simulink model "ffb_Cularis_attitudeloopclosed"  (Simulink 8.6)
settings: Solver=FixedStepAuto  SolverMode=SingleTasking  StartTime=0.0  StopTime=uavsim.simConfig.tsim  FixedStep=uavsim.simConfig.tsample_model  RelTol=1
model workspace (MAT data in the model file):
  VortexSig = Simulink.Signal
  VortexSig.DataType = 'Bus: VortexStates'
  VortexSig.Units = 'auto'
  VortexSig.Dimensions = [10 1]
  VortexSig.DimensionsMode = 'Fixed'
  VortexSig.Complexity = 'real'
  VortexSig.SampleTime = -1
  VortexSig.SamplingMode = 'auto'
  VortexSig.InitialValue = 'VortexStates_MATLABStruct_array'
undefined symbols (not defined in the file or in its folder): uavsim
libraries: aerolibtransform2 x2, aerolibutil x2, aerolibanimutils x1, uavsimBlockset_Cularis_withUAV3D x1
settings Model: Creator=mstolle  LastModifiedBy=j.bolting  ExtModeTrigDuration=100
settings SolverCC: ZcThreshold=1e-5  ZeroCrossAlgorithm=Adaptive  AlgebraicLoopSolver=LineSearch  AutoInsertRateTranBlk=on
settings DataIOCC: LimitDataPoints=off  SaveFinalState=on  SaveFormat=StructureWithTime  SignalLoggingSaveFormat=Dataset  SaveOutput=off  SaveState=on  DSMLogging=off  InspectSignalLogs=on  StateSaveName=tmp_raccel_xout
settings OptimizationCC: BlockReduction=off  OptimizeBlockIOStorage=off  BufferReuse=off  GlobalBufferReuse=off  ExpressionFolding=off  LocalBlockOutputs=off  EfficientMapNaN2IntZero=off  SimCompilerOptimization=on
settings DebuggingCC: UnderspecifiedInitializationDetection=Simplified  MergeDetectMultiDrivingBlocksExec=error  IgnoredZcDiagnostic=none  FcnCallInpInsideContextMsg=EnableAllAsError  BusObjectLabelMismatch=error
settings HardwareCC: TargetBitPerPointer=64  TargetLongLongMode=on  TargetIntDivRoundTo=Zero  TargetEndianess=LittleEndian  TargetWordSize=64  TargetHWDeviceType=MATLAB Host  ProdEqTarget=off
settings ModelReferenceCC: UpdateModelReferenceTargets=IfOutOfDate  ModelReferenceNumInstancesAllowed=Single  ModelReferenceMinAlgLoopOccurrences=on
settings SFSimCC: SFSimEcho=off
settings RTWCC: SystemTargetFile=raccel.tlc  TemplateMakefile=raccel_default_tmf  RTWVerbose=off  RTWUseSimCustomCode=on
settings CodeAppCC: GenerateComments=off  MaxIdLength=128  SimulinkBlockComments=off
settings RaccelTargetCC: ERTMultiwordTypeDef=System defined  ERTMultiwordLength=256  GeneratePreprocessorConditionals=Use local settings  ERTFirstTimeCompliant=off  MultiInstanceERTCode=off  ENABLE_SLEXEC_SSBRIDGE=0  RTWCAPIParams=on
settings ConfigComp: CovSFcnEnable=off
settings ConfigurationSet: Description=SimMechanics 2G

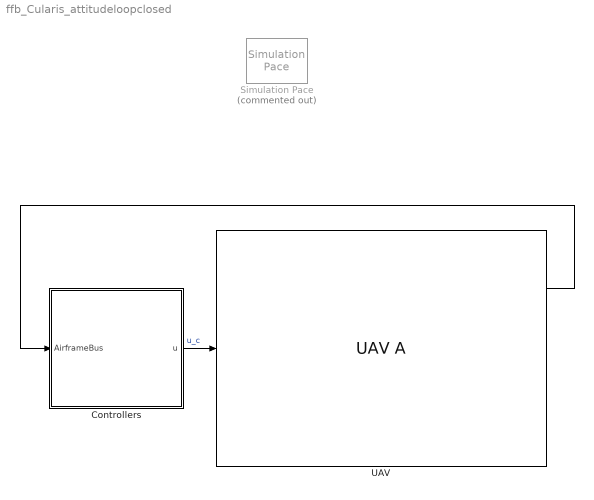
== system ffb_Cularis_attitudeloopclosed ==
  Controllers : Subsystem
  Simulation Pace : aerolibanimutils/Simulation Pace  Commented=on  SimulationPace=1  SleepMode=MATLAB Thread  OutputPaceError=off  SampleTime=-1
  UAV : uavsimBlockset_Cularis_withUAV3D/UAV A  aircraftmask_phithetapsi0=[uavsim.cularis.phithetapsi0(1:2); deg2rad(-30)]'  aircraftmask_p0_NED_m=[0 0 -50]  aircraftmask_originNED_ECEF_rrm=uavsim.originNED_ECEF_radradm  aircraftmask_pqr0=uavsim.cularis.omega0  aircraftmask_uvw0=uavsim.cularis.uvw0  aircraftmask_phithetapsi_trim=uavsim.cularis.phithetapsi0  aircraftmask_ID=1  aircraftmask_wakevortexenabled=off  aircraftmask_navigationLaw=-1  uavsim=uavsim  leaderID=0  aircraftmask_displayUAV3D=on  aircraftmask_displayVortices=off
  wires:
  UAV/1 -> Controllers/1(AirframeBus)
  Controllers/1(u) -> UAV/1  "u_c"

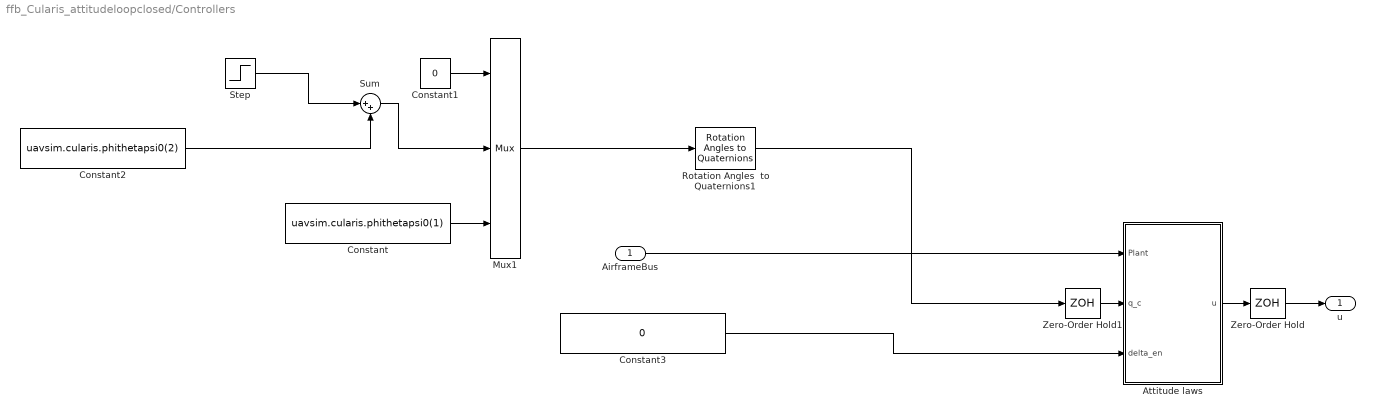
== system ffb_Cularis_attitudeloopclosed/Controllers ==
  AirframeBus : Inport
  Attitude laws : Subsystem  SystemSampleTime=uavsim.ap.hardware.dt_attitudeloops_s
  Constant : Constant  Value=uavsim.cularis.phithetapsi0(1)
  Constant1 : Constant  Value=0
  Constant2 : Constant  Value=uavsim.cularis.phithetapsi0(2)
  Constant3 : Constant  Value=0
  Mux1 : Mux  Inputs=3
  Rotation Angles  to Quaternions1 : aerolibtransform2/Rotation Angles to Quaternions  rotationOrder=ZYX
  Step : Step  Time=10  After=deg2rad(3)  SampleTime=0
  Sum : Sum  Inputs=|++
  Zero-Order Hold : ZeroOrderHold  SampleTime=uavsim.ap.tsampling_attitudelaws
  Zero-Order Hold1 : ZeroOrderHold  SampleTime=uavsim.ap.tsampling_guidancelaws
  u : Outport
  wires:
  Zero-Order Hold/1 -> u/1
  Mux1/1 -> Rotation Angles  to Quaternions1/1
  AirframeBus/1 -> Attitude laws/1(Plant)
  Attitude laws/1(u) -> Zero-Order Hold/1
  Rotation Angles  to Quaternions1/1 -> Zero-Order Hold1/1
  Zero-Order Hold1/1 -> Attitude laws/2(q_c)
  Constant1/1 -> Mux1/1
  Constant/1 -> Mux1/3
  Constant2/1 -> Sum/2
  Constant3/1 -> Attitude laws/3(delta_en)
  Step/1 -> Sum/1
  Sum/1 -> Mux1/2

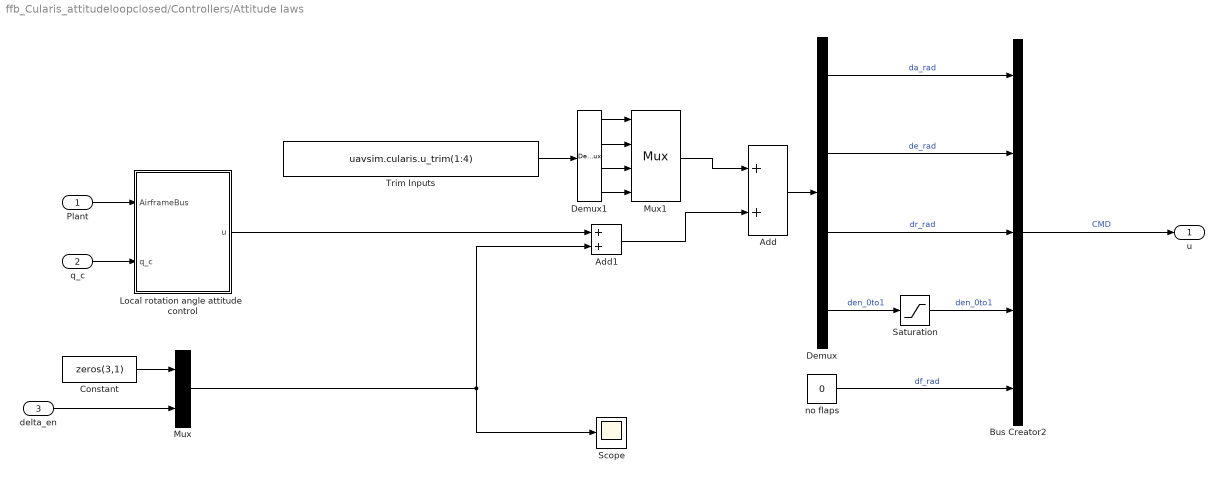
== system ffb_Cularis_attitudeloopclosed/Controllers/Attitude laws ==
  Plant : Inport  OutDataTypeStr=Bus: Airframe
  q_c : Inport  Port=2
  delta_en : Inport  Port=3
  Add : Sum
  Add1 : Sum
  Bus Creator2 : BusCreator  Inputs=5  OutDataTypeStr=Bus: CMD  NonVirtualBus=on
  Constant : Constant  Value=zeros(3,1)
  Demux : Demux
  Demux1 : Demux
  Local rotation angle attitude  control : Subsystem
  Mux : Mux  Inputs=2
  Mux1 : Mux
  Saturation : Saturate  UpperLimit=1  LowerLimit=0
  Scope : Scope
  Trim Inputs : Constant  Value=uavsim.cularis.u_trim(1:4)
  no flaps : Constant  Value=0
  u : Outport  OutDataTypeStr=Bus: CMD
  wires:
  no flaps/1 -> Bus Creator2/5  "df_rad"
  delta_en/1 -> Mux/2
  Add1/1 -> Add/2
  Mux/1 -> Scope/1, Add1/2
  Constant/1 -> Mux/1
  q_c/1 -> Local rotation angle attitude  control/2(q_c)
  Plant/1 -> Local rotation angle attitude  control/1(AirframeBus)
  Add/1 -> Demux/1
  Mux1/1 -> Add/1
  Demux/2 -> Bus Creator2/2  "de_rad"
  Demux/1 -> Bus Creator2/1  "da_rad"
  Saturation/1 -> Bus Creator2/4  "den_0to1"
  Demux/3 -> Bus Creator2/3  "dr_rad"
  Bus Creator2/1 -> u/1  "CMD"
  Local rotation angle attitude  control/1(u) -> Add1/1
  Demux/4 -> Saturation/1  "den_0to1"
  Trim Inputs/1 -> Demux1/1
  Demux1/4 -> Mux1/4
  Demux1/1 -> Mux1/1
  Demux1/3 -> Mux1/3
  Demux1/2 -> Mux1/2

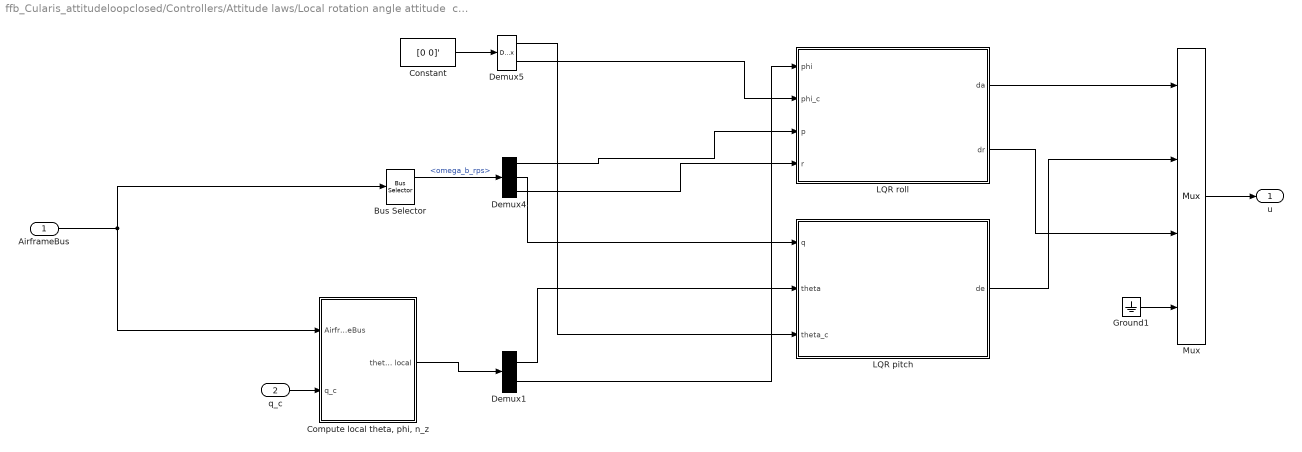
== system ffb_Cularis_attitudeloopclosed/Controllers/Attitude laws/Local rotation angle attitude  control ==
  AirframeBus : Inport  OutDataTypeStr=Bus: Airframe
  q_c : Inport  Port=2
  Bus Selector : BusSelector  OutputSignals=Kinematics.RotationalVelocity.omega_b_rps,Kinematics.Attitude.euler_rad
  "Compute local theta, phi, n_z" : Subsystem
  Constant : Constant  Value=[0 0]'
  Demux1 : Demux  Outputs=2
  Demux4 : Demux  Outputs=3
  Demux5 : Demux  Outputs=2
  Ground1 : Ground
  LQR pitch : Subsystem
  LQR roll : Subsystem
  Mux : Mux
  u : Outport
  wires:
  Ground1/1 -> Mux/4
  q_c/1 -> "Compute local theta, phi, n_z"/2(q_c)
  Mux/1 -> u/1
  Constant/1 -> Demux5/1
  Bus Selector/1 -> Demux4/1  "<omega_b_rps>"
  Demux5/2 -> LQR roll/2(phi_c)
  Demux4/1 -> LQR roll/3(p)
  Demux4/3 -> LQR roll/4(r)
  Demux5/1 -> LQR pitch/3(theta_c)
  Demux4/2 -> LQR pitch/1(q)
  LQR pitch/1(de) -> Mux/2
  LQR roll/1(da) -> Mux/1
  LQR roll/2(dr) -> Mux/3
  AirframeBus/1 -> "Compute local theta, phi, n_z"/1(AirframeBus), Bus Selector/1
  "Compute local theta, phi, n_z"/1("theta, phi local") -> Demux1/1
  Demux1/1 -> LQR pitch/2(theta)
  Demux1/2 -> LQR roll/1(phi)

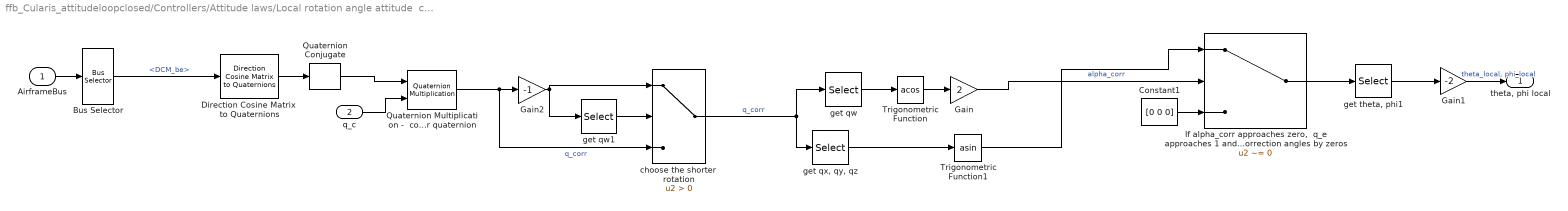
== system ffb_Cularis_attitudeloopclosed/Controllers/Attitude laws/Local rotation angle attitude  control/Compute local theta, phi, n_z ==
  AirframeBus : Inport  OutDataTypeStr=Bus: Airframe
  q_c : Inport  Port=2
  Bus Selector : BusSelector  OutputSignals=Kinematics.Attitude.DCM_be
  Constant1 : Constant  Value=[0 0 0]
  Direction Cosine Matrix  to Quaternions : aerolibtransform2/Direction Cosine Matrix  to Quaternions
  Gain : Gain  Gain=2
  Gain1 : Gain  Gain=-2
  Gain2 : Gain  Gain=-1
  "If alpha_corr approaches zero,  q_e approaches 1 and c goes to infinity.  In that case, just replace the computed  correction angles by zeros" : Switch  Criteria=u2 ~= 0
  Quaternion Conjugate : aerolibutil/Quaternion Conjugate
  Quaternion Multiplication -  compute error quaternion : aerolibutil/Quaternion Multiplication
  Trigonometric Function : Trigonometry  Operator=acos
  Trigonometric Function1 : Trigonometry  Operator=asin
  choose the shorter  rotation : Switch  Criteria=u2 > Threshold
  get qw : Selector  InputPortWidth=4  IndexOptions=Index vector (dialog)  Indices=1  OutputSizes=1
  get qw1 : Selector  InputPortWidth=4  IndexOptions=Index vector (dialog)  Indices=1  OutputSizes=1
  "get qx, qy, qz" : Selector  InputPortWidth=4  IndexOptions=Index vector (dialog)  Indices=2:4  OutputSizes=1
  "get theta, phi1" : Selector  InputPortWidth=3  IndexOptions=Index vector (dialog)  Indices=[2 1]  OutputSizes=1
  "theta, phi local" : Outport
  wires:
  AirframeBus/1 -> Bus Selector/1
  Bus Selector/1 -> Direction Cosine Matrix  to Quaternions/1  "<DCM_be>"
  q_c/1 -> Quaternion Multiplication -  compute error quaternion/2
  choose the shorter  rotation/1 -> get qw/1, "get qx, qy, qz"/1  "q_corr"
  get qw/1 -> Trigonometric Function/1
  Trigonometric Function/1 -> Gain/1
  Gain/1 -> "If alpha_corr approaches zero,  q_e approaches 1 and c goes to infinity.  In that case, just replace the computed  correction angles by zeros"/2  "alpha_corr"
  "get qx, qy, qz"/1 -> Trigonometric Function1/1
  Trigonometric Function1/1 -> "If alpha_corr approaches zero,  q_e approaches 1 and c goes to infinity.  In that case, just replace the computed  correction angles by zeros"/1
  Constant1/1 -> "If alpha_corr approaches zero,  q_e approaches 1 and c goes to infinity.  In that case, just replace the computed  correction angles by zeros"/3
  "If alpha_corr approaches zero,  q_e approaches 1 and c goes to infinity.  In that case, just replace the computed  correction angles by zeros"/1 -> "get theta, phi1"/1
  "get theta, phi1"/1 -> Gain1/1
  Quaternion Conjugate/1 -> Quaternion Multiplication -  compute error quaternion/1
  Gain1/1 -> "theta, phi local"/1  "theta_local, phi_local"
  Quaternion Multiplication -  compute error quaternion/1 -> choose the shorter  rotation/3, Gain2/1  "q_corr"
  Gain2/1 -> choose the shorter  rotation/1, get qw1/1
  get qw1/1 -> choose the shorter  rotation/2
  Direction Cosine Matrix  to Quaternions/1 -> Quaternion Conjugate/1

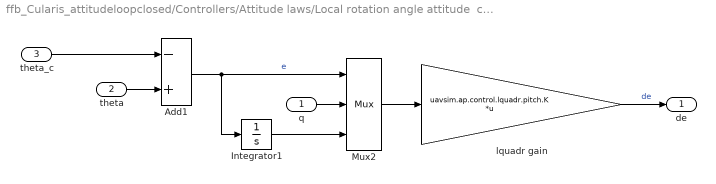
== system ffb_Cularis_attitudeloopclosed/Controllers/Attitude laws/Local rotation angle attitude  control/LQR pitch ==
  q : Inport
  theta : Inport  Port=2
  theta_c : Inport  Port=3
  Add1 : Sum  Inputs=-+
  Integrator1 : Integrator
  Mux2 : Mux  Inputs=3
  lquadr gain : Gain  Gain=uavsim.ap.control.lquadr.pitch.K  Multiplication=Matrix(K*u)
  de : Outport
  wires:
  q/1 -> Mux2/2
  Add1/1 -> Mux2/1, Integrator1/1  "e"
  theta/1 -> Add1/2
  Mux2/1 -> lquadr gain/1
  Integrator1/1 -> Mux2/3
  lquadr gain/1 -> de/1  "de"
  theta_c/1 -> Add1/1

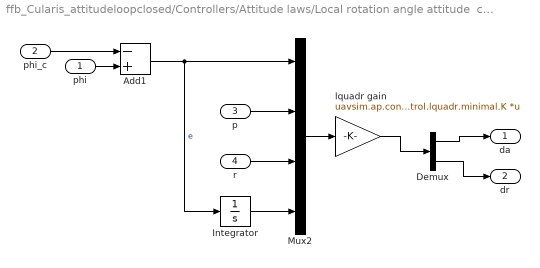
== system ffb_Cularis_attitudeloopclosed/Controllers/Attitude laws/Local rotation angle attitude  control/LQR roll ==
  phi : Inport
  phi_c : Inport  Port=2
  p : Inport  Port=3
  r : Inport  Port=4
  Add1 : Sum  Inputs=-+
  Demux : Demux  Outputs=2
  Integrator : Integrator
  Mux2 : Mux
  lquadr gain : Gain  Gain=uavsim.ap.control.lquadr.minimal.K  Multiplication=Matrix(K*u)
  da : Outport
  dr : Outport  Port=2
  wires:
  p/1 -> Mux2/2
  Demux/1 -> da/1
  Add1/1 -> Mux2/1, Integrator/1  "e"
  phi_c/1 -> Add1/1
  phi/1 -> Add1/2
  Mux2/1 -> lquadr gain/1
  Integrator/1 -> Mux2/4
  r/1 -> Mux2/3
  lquadr gain/1 -> Demux/1
  Demux/2 -> dr/1
